simulink model "PID"  (R2022a)
settings: Solver=VariableStepAuto  StartTime=0.0  StopTime=10  RelTol=1e-3
undefined symbols (not defined in the file): Kd, Ki, Kp, L, v
settings Model: Creator=leonj  LastModifiedBy=leonj

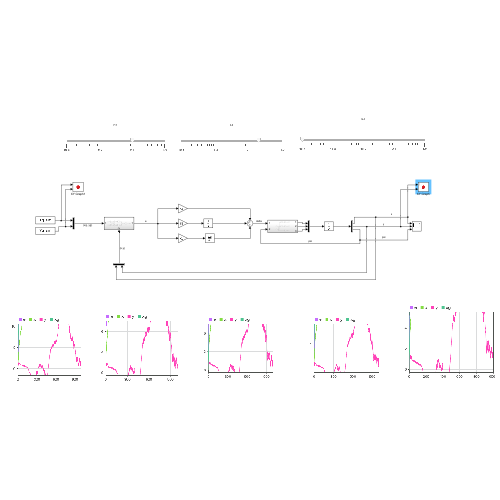
[thumbnail: Simulink's stored preview of the top-level diagram]
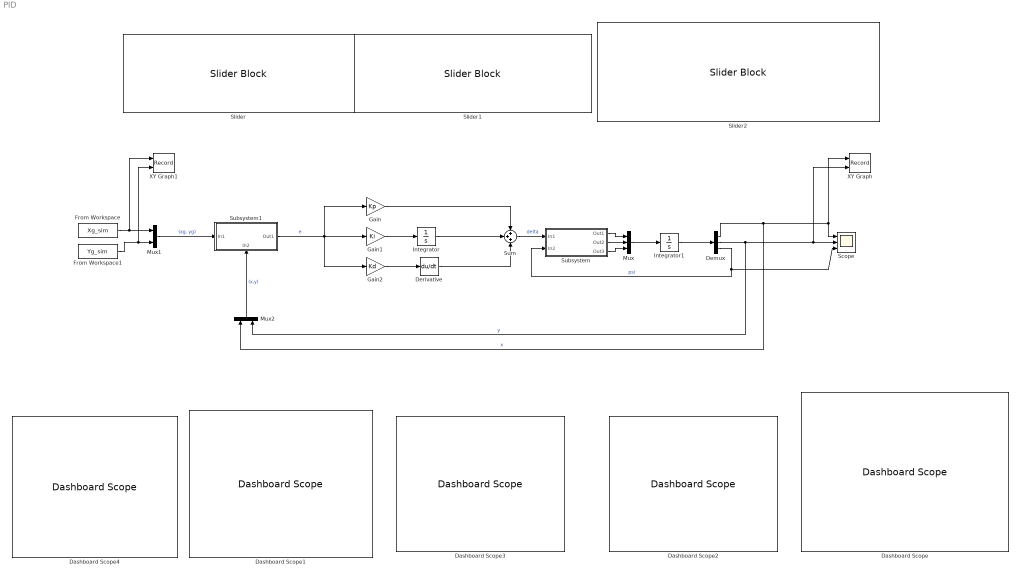
== system PID ==
  Dashboard Scope : DashboardScope  Ymin=0  Ymax=10
  Dashboard Scope1 : DashboardScope  Ymin=0  Ymax=10
  Dashboard Scope2 : DashboardScope
  Dashboard Scope3 : DashboardScope
  Dashboard Scope4 : DashboardScope
  Demux : Demux  Outputs=3
  Derivative : Derivative
  From Workspace : FromWorkspace  VariableName=Xg_sim
  From Workspace1 : FromWorkspace  VariableName=Yg_sim
  Gain : Gain  Gain=Kp
  Gain1 : Gain  Gain=Ki
  Gain2 : Gain  Gain=Kd
  Integrator : Integrator
  Integrator1 : Integrator
  Mux : Mux  Inputs=3
  Mux1 : Mux  Inputs=2
  Mux2 : Mux  Inputs=2
  Scope : Scope  NumInputPorts=3
  Slider : SliderBlock  ScaleMin=0.001  ScaleMax=1  ScaleType=Log
  Slider1 : SliderBlock  ScaleMin=0.001  ScaleMax=1  ScaleType=Log
  Slider2 : SliderBlock  ScaleMin=0.0001  ScaleMax=1  ScaleType=Log
  Subsystem : Subsystem
  Subsystem1 : Subsystem
      settings: PortSchema="{\"entries\":[{\"content\":{\"sides\":[{\"content\":{\"connectorIds\":[\"In1\"]},\"type\":\"ConnectorPlacement.EquallySpacedRectSide\",\"uuid\":\"ce90e960-11cd-4418-99a1-1b66fd5dbedd\"},{\"content\":{\"connectorIds\":[\"Out1\"],\"side\":\"RIGHT\"},\"type\":\"ConnectorPlacement.EquallySpacedRectSide\",\"uuid\":\"4009b7ba-f23e-4f4f-83b3-155686f470f1\"},{\"content\":{\"connectorIds\":[],\"side\":\"TOP\"},\"type\":\"ConnectorPlacement.EquallySpacedRectSide\",\"uuid\":\"b80a7d2e-b613-4108-bb82-78c415c4d804\"},{\"content\":{\"connectorIds\":[\"In2\"],\"side\":\"BOTTOM\"},\"type\":\"ConnectorPlacement.EquallySpacedRectSide\",\"uuid\":\"a8b029d2-5aaf-4a5a-b207-d511f0229fe7\"}]},\"type\":\"ConnectorPlacement.EquallySpacedConnector\",\"uuid\":\"491b8389-c1b4-4f5d-bd99-aaa20e708be7\"}],\"packageUris\":[\"http://schema.mathworks.com/mf0/Connector/R2020b\"],\"version\":\"1.0\"}"
  Sum : Sum  Inputs=+++
  XY Graph : Record  FileSettingsInternal="{\"entries\":[{\"content\":{\"excelSettings\":{\"content\":{},\"type\":\"Streamout.ExcelSettings\"}},\"type\":\"Streamout.FileSettingStorage\",\"uuid\":\"961bdd47-3853-4802-813f-000b40c28fd8\"}],\"packageUris\":[\"http://schema.mathworks.com/mf0/streamout_blocks/R2020a\"],\"version\":\"1.0\"}"  Layout=[1 1]  SignalsInternal="{\"entries\":[{\"content\":{\"signals\":[{\"content\":{\"blockPath\":[\"PID/XY Graph\"],\"channel\":[],\"dimensions\":[1],\"domain\":\"PID/XY Graph\",\"lineColor\":\"#a2142f\",\"plots\":[1],\"port\":1,\"sid\":[\"\"],\"signalID\":547,\"signalName\":\"x\"},\"type\":\"RecordBlkView.Signal\",\"uuid\":\"309c39d1-55fc-4469-b513-052b1a7c78a3\"},{\"content\":{\"blockPath\":[\"PID/XY Graph\"],\"channel\":[],\"dimensions\":[1],\"domain\":\"PID/XY Graph\",\"lineColor\":\"#139fff\",\"plots\":[1],\"port\":2,\"sid\":[\"\"],\"signalID\":551,\"signalName\":\"y\"},\"type\":\"RecordBlkView.Signal\",\"uuid\":\"a1542793-228a-4df4-86b2-bdca751c863d\"}]},\"type\":\"RecordBlkView.InputSignals\",\"uuid\":\"89af5198-cb0f-41c9-a47f-8b041fa5b8e7\"}],\"packageUris\":[\"http://schema.mathworks.com/mf0/streamout_blocks/R2020a\"],\"version\":\"1.0\"}"  VisualizationBindings="{\"xyplotplugin\":{\"info\":[{\"series\":[{\"bindingParametersList\":[{\"parameter\":\"X-Axis\",\"signalID\":547,\"signalName\":\"x\"},{\"parameter\":\"Y-Axis\",\"signalID\":551,\"signalName\":\"y\"}],\"seriesID\":26419}],\"subplotID\":1}]}}"  CompatibilityTag=XY
  XY Graph1 : Record  FileSettingsInternal="{\"entries\":[{\"content\":{\"excelSettings\":{\"content\":{},\"type\":\"Streamout.ExcelSettings\"}},\"type\":\"Streamout.FileSettingStorage\",\"uuid\":\"9aac4b07-02e4-4179-9e4f-172664946fb0\"}],\"packageUris\":[\"http://schema.mathworks.com/mf0/streamout_blocks/R2020a\"],\"version\":\"1.0\"}"  Layout=[1 1]  SignalsInternal="{\"entries\":[{\"content\":{\"signals\":[{\"content\":{\"blockPath\":[\"PID/XY Graph1\"],\"channel\":[],\"dimensions\":[1],\"domain\":\"PID/XY Graph1\",\"lineColor\":\"#a2142f\",\"plots\":[1],\"port\":1,\"sid\":[\"\"],\"signalID\":555,\"signalName\":\"From\\nWorkspace\"},\"type\":\"RecordBlkView.Signal\",\"uuid\":\"725d8fdc-b44a-434a-95d6-6831d6965bc6\"},{\"content\":{\"blockPath\":[\"PID/XY Graph1\"],\"channel\":[],\"dimensions\":[1],\"domain\":\"PID/XY Graph1\",\"lineColor\":\"#139fff\",\"plots\":[1],\"port\":2,\"sid\":[\"\"],\"signalID\":559,\"signalName\":\"From\\nWorkspace1\"},\"type\":\"RecordBlkView.Signal\",\"uuid\":\"3f035cd7-0344-4565-9237-90ee8e15bdab\"}]},\"type\":\"RecordBlkView.InputSignals\",\"uuid\":\"2034b807-eb45-4c31-a979-fa20235b7a37\"}],\"packageUris\":[\"http://schema.mathworks.com/mf0/streamout_blocks/R2020a\"],\"version\":\"1.0\"}"  VisualizationBindings="{\"xyplotplugin\":{\"info\":[{\"series\":[{\"bindingParametersList\":[{\"parameter\":\"X-Axis\",\"signalID\":555,\"signalName\":\"From\\nWorkspace\"},{\"parameter\":\"Y-Axis\",\"signalID\":559,\"signalName\":\"From\\nWorkspace1\"}],\"seriesID\":490}],\"subplotID\":1}]}}"  CompatibilityTag=XY
  wires:
  Gain2/1 -> Derivative/1
  Gain1/1 -> Integrator/1
  Integrator/1 -> Sum/2
  Gain/1 -> Sum/1
  Derivative/1 -> Sum/3
  Subsystem1/1(Out1) -> Gain/1, Gain1/1, Gain2/1  "e"
  Sum/1 -> Subsystem/1(In1)  "delta"
  Integrator1/1 -> Demux/1
  Demux/3 -> Subsystem/2(In2), Scope/3  "psi"
  Subsystem/3(Out3) -> Mux/3
  Subsystem/2(Out2) -> Mux/2
  Subsystem/1(Out1) -> Mux/1
  Mux/1 -> Integrator1/1
  Demux/2 -> Mux2/2, XY Graph/2, Scope/2  "y"
  Demux/1 -> Mux2/1, Scope/1, XY Graph/1  "x"
  Mux2/1 -> Subsystem1/2(In2)  "(x,y)"
  Mux1/1 -> Subsystem1/1(In1)  "(xg, yg)"
  From Workspace/1 -> XY Graph1/1, Mux1/1
  From Workspace1/1 -> XY Graph1/2, Mux1/2

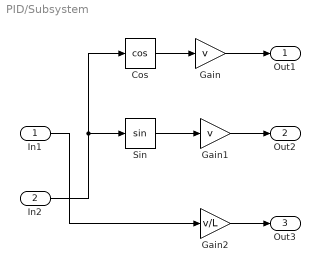
== system PID/Subsystem ==
  In1 : Inport
  In2 : Inport  Port=2
  Cos : Trigonometry  Operator=cos
  Gain : Gain  Gain=v
  Gain1 : Gain  Gain=v
  Gain2 : Gain  Gain=v/L
  Sin : Trigonometry
  Out1 : Outport
  Out2 : Outport  Port=2
  Out3 : Outport  Port=3
  wires:
  Cos/1 -> Gain/1
  Gain/1 -> Out1/1
  Sin/1 -> Gain1/1
  Gain1/1 -> Out2/1
  In2/1 -> Sin/1, Cos/1
  In1/1 -> Gain2/1
  Gain2/1 -> Out3/1

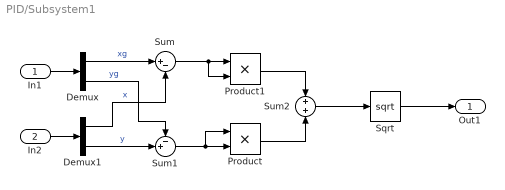
== system PID/Subsystem1 ==
  In1 : Inport
  In2 : Inport  Port=2
  Demux : Demux  Outputs=2
  Demux1 : Demux  Outputs=2
  Product : Product
  Product1 : Product
  Sqrt : Sqrt
  Sum : Sum  Inputs=|+-
  Sum1 : Sum  Inputs=-+|
  Sum2 : Sum  Inputs=+|+
  Out1 : Outport
  wires:
  Sqrt/1 -> Out1/1
  In1/1 -> Demux/1
  In2/1 -> Demux1/1
  Demux1/2 -> Sum1/2  "y"
  Demux/2 -> Sum1/1  "yg"
  Demux1/1 -> Sum/2  "x"
  Demux/1 -> Sum/1  "xg"
  Sum1/1 -> Product/1, Product/2
  Sum/1 -> Product1/2, Product1/1
  Product1/1 -> Sum2/1
  Product/1 -> Sum2/2
  Sum2/1 -> Sqrt/1
